simulink model "Sim_DB_connection"  (Simulink 10.0)
settings: Solver=FixedStepAuto  StartTime=0.0  StopTime=10.0  FixedStep=0.01  RelTol=1e-3  EnableMultiTasking=on
PreLoadFcn:
  | % Motor Parameters
  | 
  | J=0.01;     %kg*m^2
  | b=0.1;      %N*m/(rad/s)
  | K=0.01;     %V/(rad/s)
  | R=1;        %Ohm
  | L=0.5;      %H
settings Model: Creator=deastman  LastModifiedBy=Liming Gao
settings DataIOCC: LimitDataPoints=on  SaveOutput=off  SignalLogging=off  DSMLogging=off  SaveTime=off
settings OptimizationCC: ExpressionDepthLimit=2147483647  InitFltsAndDblsToZero=on
settings DebuggingCC: SolverPrmCheckMsg=warning  FcnCallInpInsideContextMsg=warning  StateNameClashWarn=warning
settings GRTTargetCC: GeneratePreprocessorConditionals=Disable all
settings ConfigComp: CovExternalEMLEnable=off

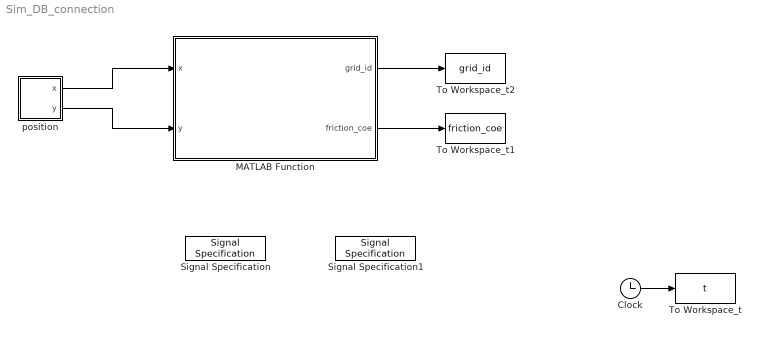
== system Sim_DB_connection ==
  Clock : Clock
  MATLAB Function : MATLAB Function  TreatAsAtomicUnit=on
  Signal Specification : SignalSpecification
  Signal Specification1 : SignalSpecification  Dimensions=1
  To Workspace_t : ToWorkspace  VariableName=t  SampleTime=-1
  To Workspace_t1 : ToWorkspace  VariableName=friction_coe  SaveFormat=Structure With Time  SampleTime=-1
  To Workspace_t2 : ToWorkspace  VariableName=grid_id  SaveFormat=Structure With Time  SampleTime=-1
      settings: Save2DSignal=2-D array (concatenate along first dimension)
  position : Subsystem
  wires:
  position/1(x) -> MATLAB Function/1(x)
  MATLAB Function/2(friction_coe) -> To Workspace_t1/1
  Clock/1 -> To Workspace_t/1
  MATLAB Function/1(grid_id) -> To Workspace_t2/1
  position/2(y) -> MATLAB Function/2(y)

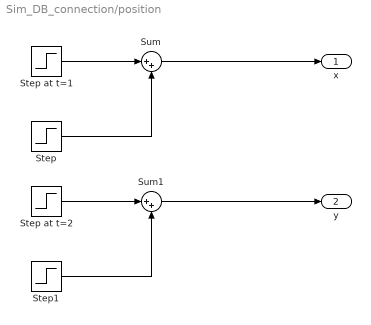
== system Sim_DB_connection/position ==
  Step : Step  Time=7  Before=1  After=3  SampleTime=0.1
  Step at t=1 : Step  Before=1  After=2  SampleTime=0.1
  Step at t=2 : Step  Before=1  After=2  SampleTime=0.1
  Step1 : Step  Time=7  Before=1  After=3  SampleTime=0.1
  Sum : Sum  Inputs=|++
  Sum1 : Sum  Inputs=|++
  x : Outport
  y : Outport  Port=2
  wires:
  Step/1 -> Sum/2
  Step at t=1/1 -> Sum/1
  Sum/1 -> x/1
  Sum1/1 -> y/1
  Step at t=2/1 -> Sum1/1
  Step1/1 -> Sum1/2

== matlab function MATLAB Function ==
  data: grid_id output double size=10000; x input double; friction_coe output double size=100; y input double
% Purpose: database query in simulink
% input: current vehicle location 
%                x: location of E,array or scalar 
%                y: location of N,
% ouput: friction coefficient
%               friction_coe:

function [grid_id,friction_coe]  = DB_query(x,y)

% Initialization
%A persistent variable is a local variable in a MATLAB function that retains 
% its value in memory between calls to the function. 
% For code generation, functions must initialize a persistent variable if it is empty. 
coder.extrinsic('database'); 
coder.extrinsic('fcn_Simulink_DB_RoadLaneGridQuery'); 
persistent flag;
persistent ip_address;
persistent database_name;
persistent username;
persistent password;
persistent driver;
persistent url;
persistent conn;
persistent results;
persistent count;
persistent sqlquery;
persistent fric;
coder.varsize('fric');
coder.varsize('friction_coe');
if isempty(flag)
    flag = 1;
    ip_address = '130.203.223.234'; %Ip address of server host
    database_name = 'nsf_roadtraffic_friction';  %%,simulator - this is the database server we will push to
    username = 'brennan'; % user name for the server
    password = 'password'; % password
    driver = 'org.postgresql.Driver'; % tells MATLAB what driver to use?
    url = ['jdbc:postgresql://' ip_address ':' num2str(5432) '/',database_name];
      
    % connect to databse
    conn = database(database_name,username,password,driver,url);
    sqlquery =['SELECT * FROM road_lane_grid where id = 2;']; % be carefule with the space
    %results = fetch(conn,sqlquery,'DataReturnFormat','numeric')
    count=1;
    fric = zeros(3,1);
end
    
%disp(get(results,'id'));
%query 
if count<10
    sqlquery =['SELECT * FROM road_lane_grid where id in (23,24,25);']; % be carefule with the space
    count = count+1;
else
    sqlquery =['SELECT * FROM road_lane_grid where id in (26,27);']; % be carefule with the space
    fric = zeros(2,1);
end
% results = fetch(conn,sqlquery,'DataReturnFormat','numeric')
% results.id; % error Attempt to extract field 'Value' from 'mxArray'.
 [~,fric]  = fcn_Simulink_DB_RoadLaneGridQuery(conn,sqlquery)
friction_coe = fric;
grid_id = 1;
